simulink library "lib_BMS_ASW"  (R2019a)
settings: Solver=VariableStepAuto  StartTime=0.0  StopTime=10.0  RelTol=1e-3
libraries: simulink x1
settings Model: Creator=wzhao  LastModifiedBy=wzhao

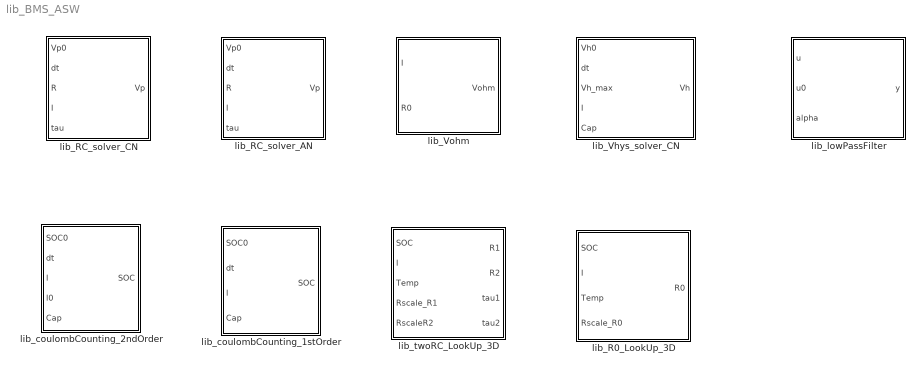
== system lib_BMS_ASW ==
  lib_R0_LookUp_3D : Subsystem  mask{Xsoc=0, Xcurrent=0, Xtemp=0, R0data=0, unitConv_R=0}
      mask prompts: Xsoc "SOC Breakpoints"; Xcurrent "Current Breakpoints"; Xtemp "Temp Breakpoints"; R0data "R0 data"; unitConv_R "Unit Conversion for R"
  lib_RC_solver_AN : Subsystem
  lib_RC_solver_CN : Subsystem  TreatAsAtomicUnit=on
  lib_Vhys_solver_CN : Subsystem  mask{Isign=0, alpha=0, unitConv_Cap=0}
      mask prompts: Isign "Current Direction"; alpha "Vhys model parameter"; unitConv_Cap "Unit Conversion for Cap"
  lib_Vohm : Subsystem
  lib_coulombCounting_1stOrder : Subsystem  mask{Isign=0, unitConv=0}
      mask prompts: Isign "Current Direction"; unitConv "Unit Conversion Factor"
  lib_coulombCounting_2ndOrder : Subsystem  mask{Isign=0, unitConv=0}
      mask prompts: Isign "Current Direction"; unitConv "Unit Conversion factor"
  lib_lowPassFilter : Subsystem
  lib_twoRC_LookUp_3D : Subsystem  mask{Xsoc=0, Xcurrent=0, Xtemp=0, R1data=0, R2data=0, tau1data=0, tau2data=0, unitConv_R=0, unitConv_tau=0}
      mask prompts: Xsoc "SOC Breakpoints"; Xcurrent "Current Breakpoints"; Xtemp "Temp Breakpoints"; R1data "R1 data"; R2data "R2 data"; tau1data "tau1 data"; tau2data "tau2 data"; unitConv_R "Unit Conversion for R"; unitConv_tau "Unit Conversion for tau"

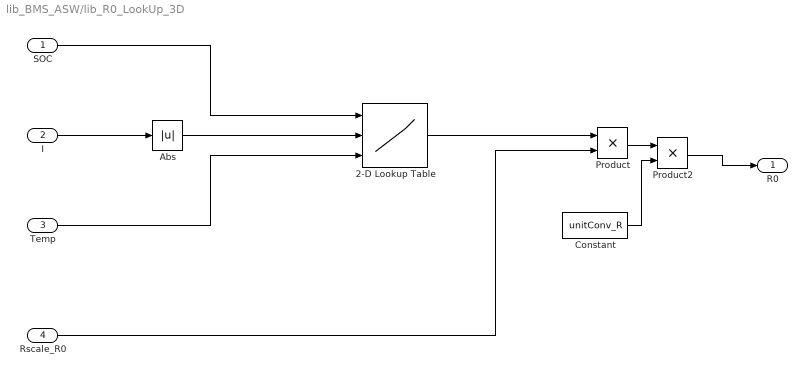
== system lib_BMS_ASW/lib_R0_LookUp_3D ==
  SOC : Inport
  I : Inport  Port=2
  Temp : Inport  Port=3
  Rscale_R0 : Inport  Port=4
  2-D Lookup Table : Lookup_n-D  NumberOfTableDimensions=3  BreakpointsForDimension1=Xsoc  BreakpointsForDimension2=Xcurrent  BreakpointsForDimension3=Xtemp  Table=R0data  InternalRulePriority=Speed  RndMeth=Simplest  InputSameDT=on
  Abs : Abs
  Constant : Constant  Value=unitConv_R
  Product : Product
  Product2 : Product
  R0 : Outport
  wires:
  Constant/1 -> Product2/2
  Product/1 -> Product2/1
  Rscale_R0/1 -> Product/2
  2-D Lookup Table/1 -> Product/1
  I/1 -> Abs/1
  Abs/1 -> 2-D Lookup Table/2
  SOC/1 -> 2-D Lookup Table/1
  Temp/1 -> 2-D Lookup Table/3
  Product2/1 -> R0/1

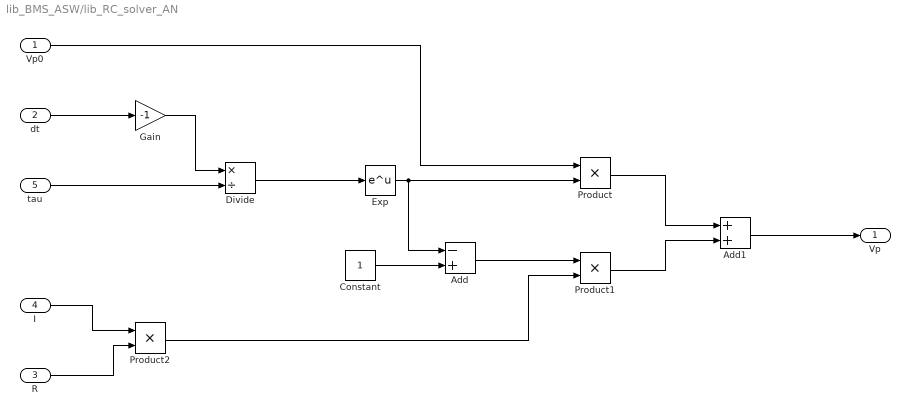
== system lib_BMS_ASW/lib_RC_solver_AN ==
  Vp0 : Inport
  dt : Inport  Port=2
  R : Inport  Port=3
  I : Inport  Port=4
  tau : Inport  Port=5
  Add : Sum  Inputs=-+
  Add1 : Sum
  Constant : Constant
  Divide : Product  Inputs=*/
  Exp : Math  SaturateOnIntegerOverflow=on
  Gain : Gain  Gain=-1
  Product : Product
  Product1 : Product
  Product2 : Product
  Vp : Outport
  wires:
  dt/1 -> Gain/1
  Gain/1 -> Divide/1
  tau/1 -> Divide/2
  Divide/1 -> Exp/1
  Exp/1 -> Add/1, Product/2
  Vp0/1 -> Product/1
  Constant/1 -> Add/2
  Add/1 -> Product1/1
  Product/1 -> Add1/1
  Product1/1 -> Add1/2
  Add1/1 -> Vp/1
  I/1 -> Product2/1
  R/1 -> Product2/2
  Product2/1 -> Product1/2

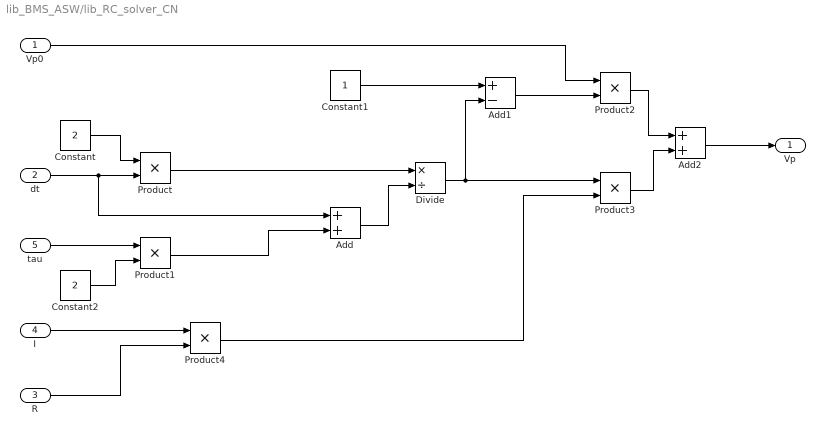
== system lib_BMS_ASW/lib_RC_solver_CN ==
  Vp0 : Inport
  dt : Inport  Port=2
  R : Inport  Port=3
  I : Inport  Port=4
  tau : Inport  Port=5
  Add : Sum
  Add1 : Sum  Inputs=+-
  Add2 : Sum
  Constant : Constant  Value=2
  Constant1 : Constant
  Constant2 : Constant  Value=2
  Divide : Product  Inputs=*/
  Product{,1..4} (5 alike) : Product
  Vp : Outport
  wires:
  dt/1 -> Product/2, Add/1
  tau/1 -> Product1/1
  Constant2/1 -> Product1/2
  Product1/1 -> Add/2
  Constant/1 -> Product/1
  Product/1 -> Divide/1
  Add/1 -> Divide/2
  Constant1/1 -> Add1/1
  Divide/1 -> Add1/2, Product3/1
  Add1/1 -> Product2/2
  Vp0/1 -> Product2/1
  Product2/1 -> Add2/1
  Product3/1 -> Add2/2
  Add2/1 -> Vp/1
  I/1 -> Product4/1
  R/1 -> Product4/2
  Product4/1 -> Product3/2

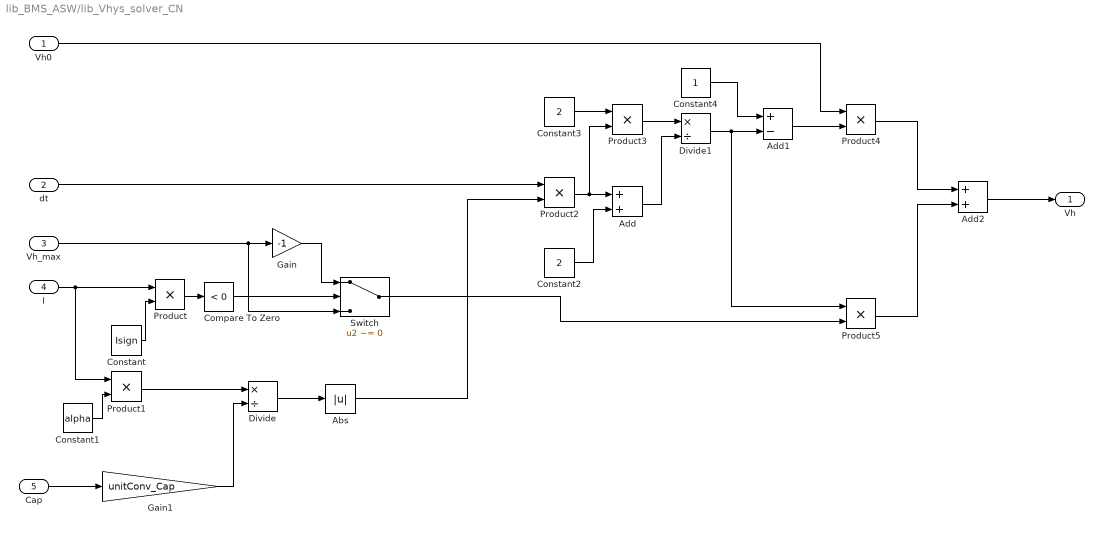
== system lib_BMS_ASW/lib_Vhys_solver_CN ==
  Vh0 : Inport
  dt : Inport  Port=2
  Vh_max : Inport  Port=3
  I : Inport  Port=4
  Cap : Inport  Port=5
  Abs : Abs
  Add : Sum
  Add1 : Sum  Inputs=+-
  Add2 : Sum
  Compare To Zero : simulink/Logic and Bit Operations/Compare To Zero  relop=<  OutDataTypeStr=boolean
  Constant : Constant  Value=Isign
  Constant1 : Constant  Value=alpha
  Constant2 : Constant  Value=2
  Constant3 : Constant  Value=2
  Constant4 : Constant
  Divide : Product  Inputs=*/
  Divide1 : Product  Inputs=*/
  Gain : Gain  Gain=-1
  Gain1 : Gain  Gain=unitConv_Cap
  Product{,1..5} (6 alike) : Product
  Switch : Switch  Criteria=u2 ~= 0
  Vh : Outport
  wires:
  I/1 -> Product1/1, Product/1
  Constant/1 -> Product/2
  Product/1 -> Compare To Zero/1
  Compare To Zero/1 -> Switch/2
  Vh_max/1 -> Switch/3, Gain/1
  Gain/1 -> Switch/1
  Constant1/1 -> Product1/2
  Product1/1 -> Divide/1
  Cap/1 -> Gain1/1
  Gain1/1 -> Divide/2
  Divide/1 -> Abs/1
  Switch/1 -> Product5/2
  dt/1 -> Product2/1
  Product2/1 -> Product3/2, Add/1
  Constant2/1 -> Add/2
  Constant3/1 -> Product3/1
  Product3/1 -> Divide1/1
  Add/1 -> Divide1/2
  Divide1/1 -> Product5/1, Add1/2
  Constant4/1 -> Add1/1
  Add1/1 -> Product4/2
  Vh0/1 -> Product4/1
  Abs/1 -> Product2/2
  Product4/1 -> Add2/1
  Product5/1 -> Add2/2
  Add2/1 -> Vh/1

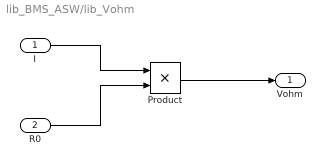
== system lib_BMS_ASW/lib_Vohm ==
  I : Inport
  R0 : Inport  Port=2
  Product : Product
  Vohm : Outport
  wires:
  I/1 -> Product/1
  R0/1 -> Product/2
  Product/1 -> Vohm/1

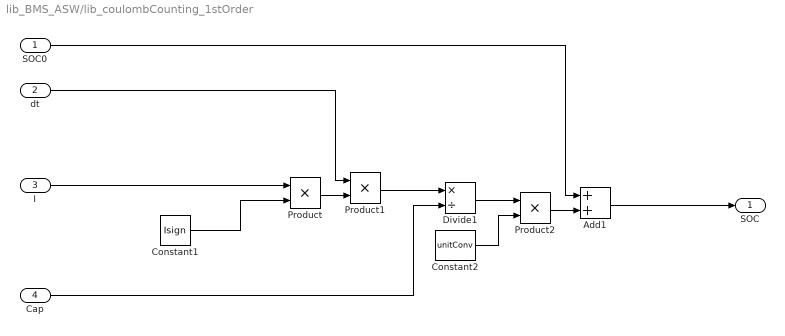
== system lib_BMS_ASW/lib_coulombCounting_1stOrder ==
  SOC0 : Inport
  dt : Inport  Port=2
  I : Inport  Port=3
  Cap : Inport  Port=4
  Add1 : Sum
  Constant1 : Constant  Value=Isign  SampleTime=-1
  Constant2 : Constant  Value=unitConv  SampleTime=-1
  Divide1 : Product  Inputs=*/
  Product : Product
  Product1 : Product
  Product2 : Product
  SOC : Outport
  wires:
  Add1/1 -> SOC/1
  SOC0/1 -> Add1/1
  Product2/1 -> Add1/2
  Constant2/1 -> Product2/2
  Divide1/1 -> Product2/1
  Cap/1 -> Divide1/2
  Product1/1 -> Divide1/1
  dt/1 -> Product1/1
  Product/1 -> Product1/2
  Constant1/1 -> Product/2
  I/1 -> Product/1

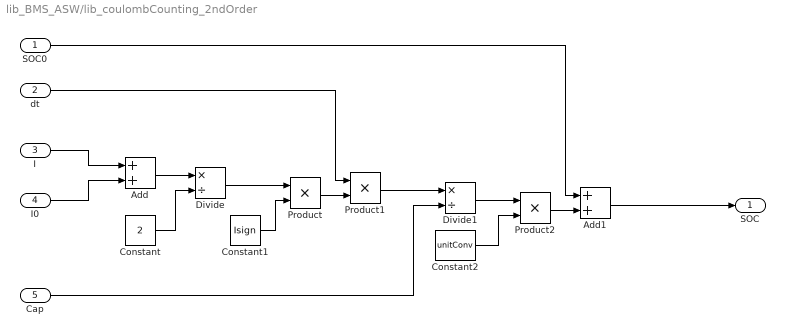
== system lib_BMS_ASW/lib_coulombCounting_2ndOrder ==
  SOC0 : Inport
  dt : Inport  Port=2
  I : Inport  Port=3
  I0 : Inport  Port=4
  Cap : Inport  Port=5
  Add : Sum
  Add1 : Sum
  Constant : Constant  Value=2  SampleTime=-1
  Constant1 : Constant  Value=Isign  SampleTime=-1
  Constant2 : Constant  Value=unitConv  SampleTime=-1
  Divide : Product  Inputs=*/
  Divide1 : Product  Inputs=*/
  Product : Product
  Product1 : Product
  Product2 : Product
  SOC : Outport
  wires:
  I/1 -> Add/1
  I0/1 -> Add/2
  Add/1 -> Divide/1
  Constant/1 -> Divide/2
  Divide/1 -> Product/1
  Constant1/1 -> Product/2
  Product/1 -> Product1/2
  dt/1 -> Product1/1
  Product1/1 -> Divide1/1
  Cap/1 -> Divide1/2
  Divide1/1 -> Product2/1
  Constant2/1 -> Product2/2
  Product2/1 -> Add1/2
  SOC0/1 -> Add1/1
  Add1/1 -> SOC/1

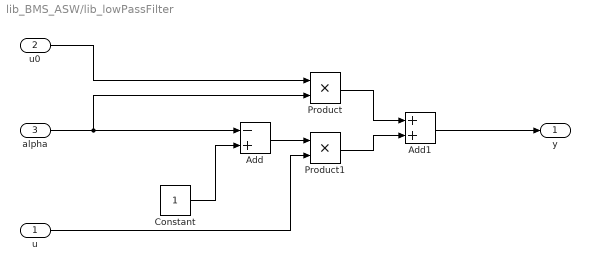
== system lib_BMS_ASW/lib_lowPassFilter ==
  u : Inport
  u0 : Inport  Port=2
  alpha : Inport  Port=3
  Add : Sum  Inputs=-+
  Add1 : Sum
  Constant : Constant
  Product : Product
  Product1 : Product
  y : Outport
  wires:
  u0/1 -> Product/1
  alpha/1 -> Add/1, Product/2
  Constant/1 -> Add/2
  Add/1 -> Product1/1
  u/1 -> Product1/2
  Product/1 -> Add1/1
  Product1/1 -> Add1/2
  Add1/1 -> y/1

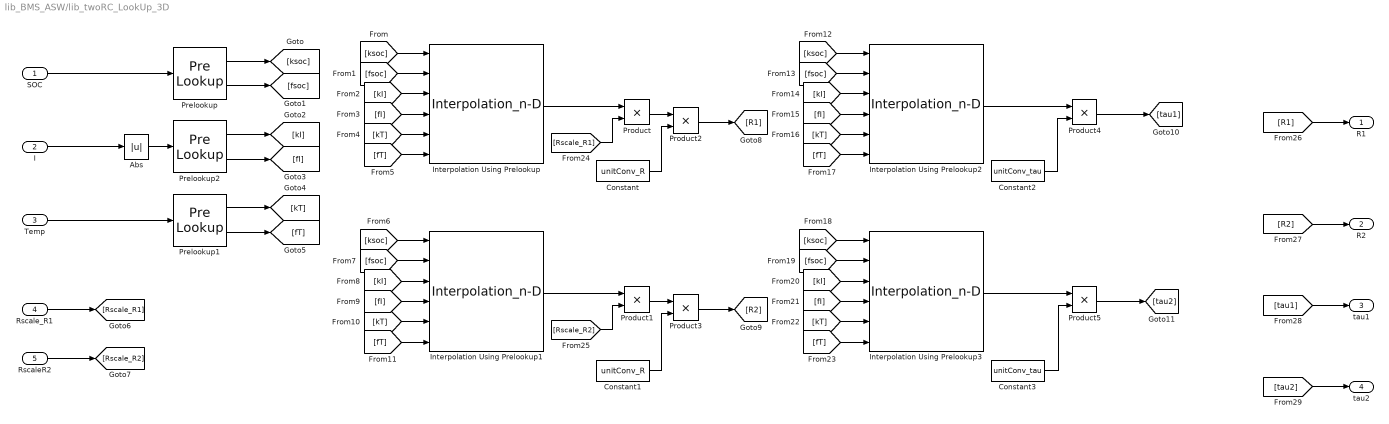
== system lib_BMS_ASW/lib_twoRC_LookUp_3D ==
  SOC : Inport
  I : Inport  Port=2
  Temp : Inport  Port=3
  Rscale_R1 : Inport  Port=4
  RscaleR2 : Inport  Port=5
  Abs : Abs
  Constant : Constant  Value=unitConv_R
  Constant1 : Constant  Value=unitConv_R
  Constant2 : Constant  Value=unitConv_tau
  Constant3 : Constant  Value=unitConv_tau
  Interpolation Using Prelookup : Interpolation_n-D  NumberOfTableDimensions=3  Table=R1data  ExtrapMethod=Clip  InternalRulePriority=Speed
      settings: InputPortMap=u0,u1,u2,u3,u4,u5
  Interpolation Using Prelookup1 : Interpolation_n-D  NumberOfTableDimensions=3  Table=R2data  ExtrapMethod=Clip  InternalRulePriority=Speed
      settings: InputPortMap=u0,u1,u2,u3,u4,u5
  Interpolation Using Prelookup2 : Interpolation_n-D  NumberOfTableDimensions=3  Table=tau1data  ExtrapMethod=Clip  InternalRulePriority=Speed
      settings: InputPortMap=u0,u1,u2,u3,u4,u5
  Interpolation Using Prelookup3 : Interpolation_n-D  NumberOfTableDimensions=3  Table=tau2data  ExtrapMethod=Clip  InternalRulePriority=Speed
      settings: InputPortMap=u0,u1,u2,u3,u4,u5
  Prelookup : PreLookup  BreakpointsData=Xsoc  ExtrapMethod=Linear
  Prelookup1 : PreLookup  BreakpointsData=Xtemp  ExtrapMethod=Linear
  Prelookup2 : PreLookup  BreakpointsData=Xcurrent  ExtrapMethod=Linear
  Product{,1..5} (6 alike) : Product
  R1 : Outport
  R2 : Outport  Port=2
  tau1 : Outport  Port=3
  tau2 : Outport  Port=4
  wires:
  SOC/1 -> Prelookup/1
  I/1 -> Abs/1
  Temp/1 -> Prelookup1/1
  Abs/1 -> Prelookup2/1
  Prelookup/1 -> [ksoc]
  Prelookup/2 -> [fsoc]
  Prelookup2/1 -> [kI]
  Prelookup2/2 -> [fI]
  Prelookup1/1 -> [kT]
  Prelookup1/2 -> [fT]
  [ksoc] -> Interpolation Using Prelookup/1
  [fsoc] -> Interpolation Using Prelookup/2
  [kI] -> Interpolation Using Prelookup/3
  [fI] -> Interpolation Using Prelookup/4
  [kT] -> Interpolation Using Prelookup/5
  [fT] -> Interpolation Using Prelookup/6
  [kT] -> Interpolation Using Prelookup1/5
  [fT] -> Interpolation Using Prelookup1/6
  [fsoc] -> Interpolation Using Prelookup1/2
  [ksoc] -> Interpolation Using Prelookup1/1
  [fI] -> Interpolation Using Prelookup1/4
  [kI] -> Interpolation Using Prelookup1/3
  [kT] -> Interpolation Using Prelookup2/5
  [fT] -> Interpolation Using Prelookup2/6
  [fsoc] -> Interpolation Using Prelookup2/2
  [ksoc] -> Interpolation Using Prelookup2/1
  [fI] -> Interpolation Using Prelookup2/4
  [kI] -> Interpolation Using Prelookup2/3
  [kT] -> Interpolation Using Prelookup3/5
  [fT] -> Interpolation Using Prelookup3/6
  [fsoc] -> Interpolation Using Prelookup3/2
  [ksoc] -> Interpolation Using Prelookup3/1
  [fI] -> Interpolation Using Prelookup3/4
  [kI] -> Interpolation Using Prelookup3/3
  Rscale_R1/1 -> [Rscale_R1]
  RscaleR2/1 -> [Rscale_R2]
  Interpolation Using Prelookup/1 -> Product/1
  [Rscale_R1] -> Product/2
  Interpolation Using Prelookup1/1 -> Product1/1
  [Rscale_R2] -> Product1/2
  Product/1 -> Product2/1
  Constant/1 -> Product2/2
  Product1/1 -> Product3/1
  Constant1/1 -> Product3/2
  Interpolation Using Prelookup2/1 -> Product4/1
  Constant2/1 -> Product4/2
  Interpolation Using Prelookup3/1 -> Product5/1
  Constant3/1 -> Product5/2
  Product2/1 -> [R1]
  Product3/1 -> [R2]
  Product4/1 -> [tau1]
  Product5/1 -> [tau2]
  [R1] -> R1/1
  [tau1] -> tau1/1
  [tau2] -> tau2/1
  [R2] -> R2/1
